simulink model "lab9model1"  (R2023a)
settings: Solver=VariableStepAuto  StartTime=0.0  StopTime=0.0  RelTol=1e-3
settings Model: Creator=losingmysanity  LastModifiedBy=losingmysanity

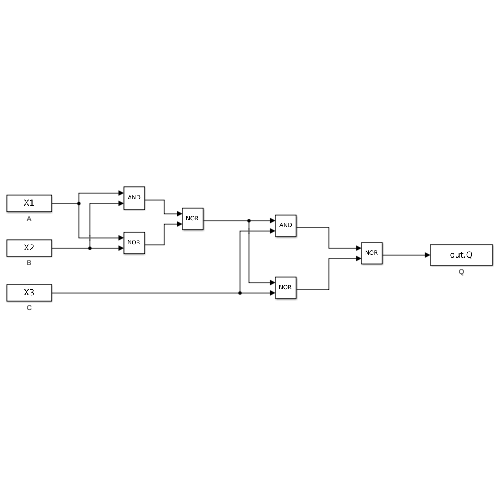
[thumbnail: Simulink's stored preview of the top-level diagram]
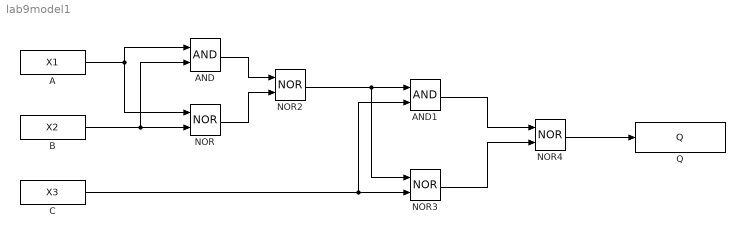
== system lab9model1 ==
  A : FromWorkspace  VariableName=X1
  AND : Logic  AllPortsSameDT=off  OutDataTypeStr=boolean
  AND1 : Logic  AllPortsSameDT=off  OutDataTypeStr=boolean
  B : FromWorkspace  VariableName=X2
  C : FromWorkspace  VariableName=X3
  NOR{,2..4} (4 alike) : Logic  Operator=NOR  AllPortsSameDT=off  OutDataTypeStr=boolean
  Q : ToWorkspace  VariableName=Q  SaveFormat=Timeseries  SampleTime=-1
  wires:
  A/1 -> NOR/1, AND/1
  B/1 -> AND/2, NOR/2
  AND/1 -> NOR2/1
  NOR/1 -> NOR2/2
  NOR2/1 -> NOR3/1, AND1/1
  C/1 -> NOR3/2, AND1/2
  AND1/1 -> NOR4/1
  NOR3/1 -> NOR4/2
  NOR4/1 -> Q/1
